simulink model "differentiator"  (Simulink 4.00)
settings: Solver=ode45  StartTime=0.0  StopTime=tfinal  MaxStep=0.01  RelTol=1e-3
values from neighbouring files (symbols this model uses):
  tau_diff = 0.02    [CreatVariablesForPlotting.m]    (also in plot_states.m; setup_for_plotting.m)
settings Model: LastModifiedBy=rajamani  OutputOption=SpecifiedOutputTimes  OutputTimes=t

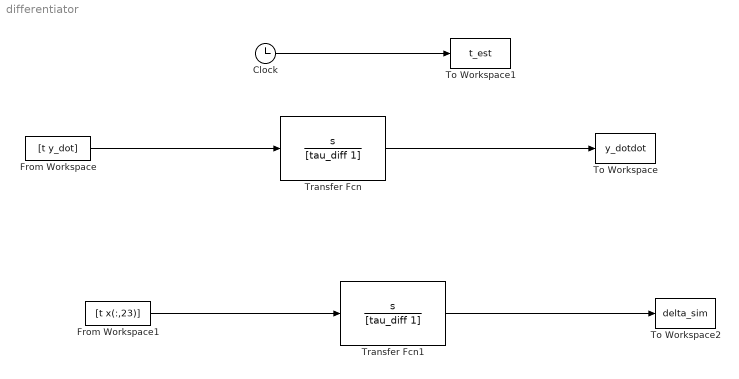
== system differentiator ==
  Clock : Clock
      settings: DisplayTime=off  Decimation=10
  From Workspace : FromWorkspace  VariableName=[t y_dot]  SampleTime=0  OutputAfterFinalValue=Extrapolation
  From Workspace1 : FromWorkspace  VariableName=[t x(:,23)]  SampleTime=0  OutputAfterFinalValue=Extrapolation
  To Workspace : ToWorkspace  VariableName=y_dotdot  SampleTime=-1  SaveFormat=Array
  To Workspace1 : ToWorkspace  VariableName=t_est  SampleTime=-1  SaveFormat=Array
  To Workspace2 : ToWorkspace  VariableName=delta_sim  SampleTime=-1  SaveFormat=Array
  Transfer Fcn : TransferFcn  Numerator=[1 0]  Denominator=[tau_diff 1]  AbsoluteTolerance=auto  Realization=auto
  Transfer Fcn1 : TransferFcn  Numerator=[1 0]  Denominator=[tau_diff 1]  AbsoluteTolerance=auto  Realization=auto
  wires:
  From Workspace/1 -> Transfer Fcn/1
  Transfer Fcn/1 -> To Workspace/1
  Clock/1 -> To Workspace1/1
  From Workspace1/1 -> Transfer Fcn1/1
  Transfer Fcn1/1 -> To Workspace2/1
